simulink model "receiver_1"  (R2023a)
settings: Solver=FixedStepAuto  StartTime=0.0  StopTime=10.0  RelTol=1e-3
undefined symbols (not defined in the file): Data_Display, M, receiver_nihar, SC_1_DC_0
libraries: androiduilib x5, androidaudiovideolib x2, androidcommunicationlib x2
settings Model: Creator=mohit  LastModifiedBy=mohit
settings OptimizationCC: EnhancedBackFolding=on  PassReuseOutputArgsAs=Individual arguments  ZeroExternalMemoryAtStartup=off  ZeroInternalMemoryAtStartup=off  MaxStackSize=64  OptimizeBlockOrder=speed  DifferentSizesBufferReuse=on  OptimizationCustomize=off  EfficientTunableParamExpr=on
settings DebuggingCC: ParameterTunabilityLossMsg=error
settings HardwareCC: ProdBitPerLong=64  ProdLargestAtomicInteger=LongLong  ProdLargestAtomicFloat=Double  ProdLongLongMode=on  ProdHWDeviceType=ARM Compatible->ARM 64-bit (LP64)  UseEmbeddedCoderFeatures=off  UseSimulinkCoderFeatures=off
settings SFSimCC: MATLABDynamicMemAlloc=off
settings RTWCC: Description=Embedded Coder  SystemTargetFile=ert.tlc  HardwareBoard=Android Device (64bit)  TLCOptions="-aInlineSetEventsForThisBaseRateFcn=TLC_FALSE -aSuppressMultiTaskScheduler=TLC_FALSE  -aRateBasedStepFcn=0"  TemplateMakefile=ert_default_tmf  RTWVerbose=off  Toolchain=Android SDK/NDK Tools
settings CodeAppCC: ForceParamTrailComments=on  IgnoreCustomStorageClasses=off  OperatorAnnotations=on  SimulinkDataObjDesc=on  SFDataObjDesc=on  InsertBlockDesc=on
settings ERTTargetCC: SupportNonInlinedSFcns=on

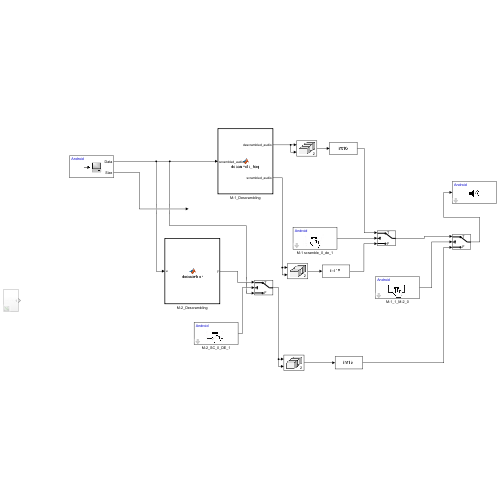
[thumbnail: Simulink's stored preview of the top-level diagram]
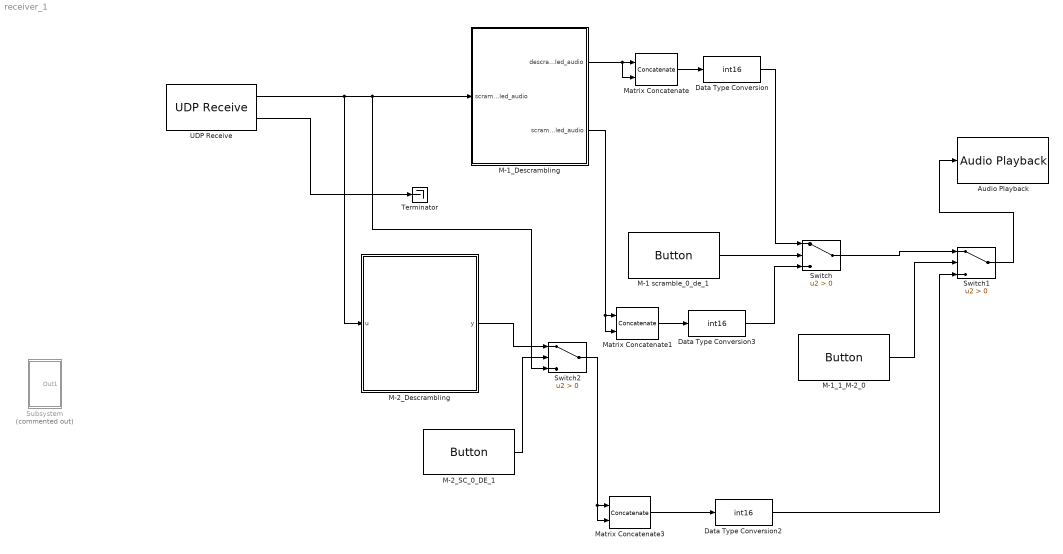
== system receiver_1 ==
  Audio Playback : androidaudiovideolib/Audio Playback  SampleFreq=44100  AudioSamplingFreq=44100  SampleTime=0.1  DeviceStr=0  QueueDuration=0  BlockPlatform=Android
  Data Type Conversion : DataTypeConversion  OutDataTypeStr=int16  SaturateOnIntegerOverflow=off  RndMeth=Floor
  Data Type Conversion2 : DataTypeConversion  OutDataTypeStr=int16  SaturateOnIntegerOverflow=off  RndMeth=Floor
  Data Type Conversion3 : DataTypeConversion  OutDataTypeStr=int16  SaturateOnIntegerOverflow=off  RndMeth=Floor
  M-1 scramble_0_de_1 : androiduilib/Button  ButtonState=Not pressed  ButtonId=receiver_nihar/M-1_scramble_0_de_1  State=off  SampleTime=0.1  BlockPlatform=Android
  M-1_1_M-2_0 : androiduilib/Button  ButtonState=Not pressed  ButtonId=receiver_nihar/M-1_1_M-2_0  State=off  SampleTime=0.1  BlockPlatform=Android
  M-1_Descrambling : MATLAB Function  TreatAsAtomicUnit=on
  M-2_Descrambling : MATLAB Function  TreatAsAtomicUnit=on
  M-2_SC_0_DE_1 : androiduilib/Button  ButtonState=Not pressed  ButtonId=receiver_nihar/M-2_SC_0_DE_1  State=off  SampleTime=0.1  BlockPlatform=Android
  Matrix Concatenate : Concatenate  Mode=Multidimensional array  ConcatenateDimension=2
  Matrix Concatenate1 : Concatenate  Mode=Multidimensional array  ConcatenateDimension=2
  Matrix Concatenate3 : Concatenate  Mode=Multidimensional array  ConcatenateDimension=2
  Subsystem : Subsystem  Commented=on
  Switch : Switch  Criteria=u2 > Threshold  SaturateOnIntegerOverflow=off  InputSameDT=off
  Switch1 : Switch  Criteria=u2 > Threshold  SaturateOnIntegerOverflow=off  InputSameDT=off
  Switch2 : Switch  Criteria=u2 > Threshold  SaturateOnIntegerOverflow=off  InputSameDT=off
  Terminator : Terminator
  UDP Receive : androidcommunicationlib/UDP Receive  localURL='0.0.0.0'  localPort=35000  remoteURL='0.0.0.0'  remotePort=-1  recvBufferSize=8192  signalDatatype=int16  dims=2205  isVarSize=off  showBlockingTime=off  blockingTime=0  sampletime=0.05  blockPlatform=Android
  wires:
  UDP Receive/2 -> Terminator/1
  M-1_Descrambling/1(descrambled_audio) -> Matrix Concatenate/2, Matrix Concatenate/1
  Matrix Concatenate/1 -> Data Type Conversion/1
  M-1 scramble_0_de_1/1 -> Switch/2
  UDP Receive/1 -> Switch2/3, M-1_Descrambling/1("scrambled_audio "), M-2_Descrambling/1(u)
  M-1_Descrambling/2(scrambled_audio) -> Matrix Concatenate1/2, Matrix Concatenate1/1
  Data Type Conversion/1 -> Switch/1
  Matrix Concatenate3/1 -> Data Type Conversion2/1
  Matrix Concatenate1/1 -> Data Type Conversion3/1
  Data Type Conversion3/1 -> Switch/3
  Switch/1 -> Switch1/1
  Switch1/1 -> Audio Playback/1
  M-1_1_M-2_0/1 -> Switch1/2
  M-2_Descrambling/1(y) -> Switch2/1
  M-2_SC_0_DE_1/1 -> Switch2/2
  Switch2/1 -> Matrix Concatenate3/2, Matrix Concatenate3/1
  Data Type Conversion2/1 -> Switch1/3

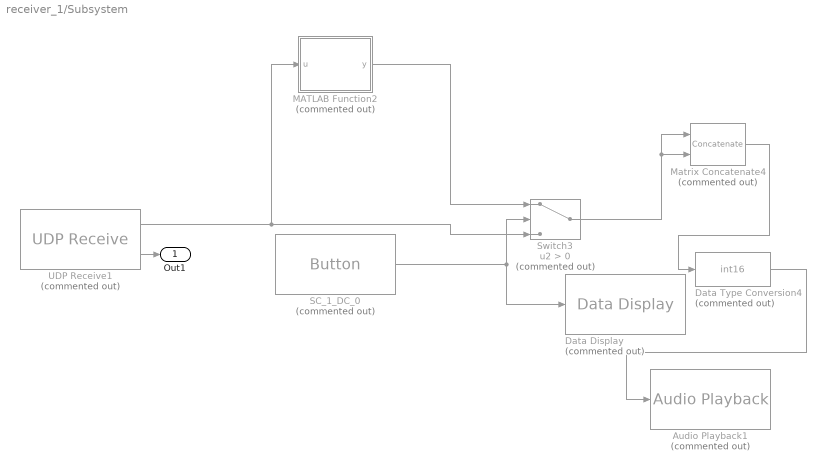
== system receiver_1/Subsystem ==
  Audio Playback1 : androidaudiovideolib/Audio Playback  Commented=on  SampleFreq=44100  AudioSamplingFreq=44100  SampleTime=0.1  DeviceStr=0  QueueDuration=0  BlockPlatform=Android
  Data Display : androiduilib/Data Display  Commented=on  DataDisplayId=receiver_nihar/Data_Display  Format=Float  Precision=6  SimulateUsing=Code generation  blockPlatform=Android
  Data Type Conversion4 : DataTypeConversion  Commented=on  OutDataTypeStr=int16  SaturateOnIntegerOverflow=off  RndMeth=Floor
  MATLAB Function2 : MATLAB Function  Commented=on  TreatAsAtomicUnit=on
  Matrix Concatenate4 : Concatenate  Commented=on  Mode=Multidimensional array  ConcatenateDimension=2
  SC_1_DC_0 : androiduilib/Button  Commented=on  ButtonState=Not pressed  ButtonId=receiver_nihar/SC_1_DC_0  State=off  SampleTime=0.1  BlockPlatform=Android
  Switch3 : Switch  Commented=on  Criteria=u2 > Threshold  SaturateOnIntegerOverflow=off  InputSameDT=off
  UDP Receive1 : androidcommunicationlib/UDP Receive  Commented=on  localURL='0.0.0.0'  localPort=35000  remoteURL='0.0.0.0'  remotePort=-1  recvBufferSize=8192  signalDatatype=int16  dims=2205  isVarSize=off  showBlockingTime=off  blockingTime=0  sampletime=0.05  blockPlatform=Android
  Out1 : Outport
  wires:
  Data Type Conversion4/1 -> Audio Playback1/1
  Switch3/1 -> Matrix Concatenate4/1, Matrix Concatenate4/2
  SC_1_DC_0/1 -> Data Display/1, Switch3/2
  UDP Receive1/1 -> Switch3/3, MATLAB Function2/1(u)
  UDP Receive1/2 -> Out1/1
  Matrix Concatenate4/1 -> Data Type Conversion4/1
  MATLAB Function2/1(y) -> Switch3/1

== matlab function receiver_1/M-2_Descrambling ==
  data: u input; y output
function y = descrambler(u)
    % Extract the first channel of the input matrix (assuming u is Nx2)
    u = u(:,1);

    % Define the bucket size
    bucketSize = 20;

    % Perform FFT on the entire signal
    fftResult = fft(u);
    
    % Number of buckets in the entire signal
    numBuckets = floor(length(fftResult) / bucketSize);

    % Subtract the exact noise added during scrambling
    for i = 1:numBuckets
        % Define the range of indices for this bucket
        bucketStartIdx = (i-1) * bucketSize + 1;
        bucketEndIdx = bucketStartIdx + bucketSize - 1;

        % Remove noise from each element in the bucket
        for idx = bucketStartIdx:bucketEndIdx
            noise = (idx +10) * 1e6;  % Calculate noise as index * 10,00,000
            fftResult(idx) = fftResult(idx) - noise;  % Remove noise from positive frequency
            fftResult(end - idx + 2) = fftResult(end - idx + 2) - noise;  % Remove noise from negative frequency
        end
    end

    % Handle any remaining elements outside of full buckets
    if mod(length(fftResult), bucketSize) ~= 0
        remainingStart = numBuckets * bucketSize + 1;
        for idx = remainingStart:length(fftResult)
            noise = (idx+10) * 1e6;  % Calculate noise as index * 10,00,000
            fftResult(idx) = fftResult(idx) - noise;  % Remove noise from positive frequency
            fftResult(end - idx + 2) = fftResult(end - idx + 2) - noise;  % Remove noise from negative frequency
        end
    end

    % Enforce conjugate symmetry on fftResult to ensure real output from ifft
    N = length(fftResult);
    fftResult(2:N/2) = conj(fftResult(N:-1:N/2+2));

    % Perform the inverse FFT to get the descrambled time-domain signal
    descrambledChannel = ifft(fftResult);

    % Take the real part to ensure the output is real-valued
    y = real(descrambledChannel);
end

== matlab function receiver_1/M-1_Descrambling ==
  data: scrambled_audio input; descrambled_audio output; scrambled_audio output
function [descrambled_audio,scrambled_audio] = descramble_freq(scrambled_audio)
    % Descramble the scrambled audio input in the frequency domain using the same seed
    % scrambled_audio: [nx2] scrambled audio array
    % seed: The same integer seed used during scrambling
    seed=123;
    % Pre-allocate descrambled_audio array
    descrambled_audio = zeros(size(scrambled_audio));

    % Set the random seed to regenerate the same permutation
    rng(seed, 'twister');
    
    % Generate the same random permutation as scrambling
    n = size(scrambled_audio, 1);
    swap_indices = randperm(n);
    scrambled_audio=scrambled_audio(:,1);
    % Apply FFT to each channel separately
    scrambled_freq_left = fft(scrambled_audio(:,1));
    %scrambled_freq_right = fft(scrambled_audio(:,2));

    % Reverse the swapping using the inverse of swap_indices
    [~, inverse_indices] = sort(swap_indices);
    descrambled_freq_left = scrambled_freq_left(inverse_indices);
    %descrambled_freq_right = scrambled_freq_right(inverse_indices);

    % Convert back to time domain
    descrambled_audio(:,1) = real(ifft(descrambled_freq_left));
    %descrambled_audio(:,2) = real(ifft(descrambled_freq_right));
end

== matlab function receiver_1/Subsystem/MATLAB Function2 ==
  data: u input; y output
function y = descrambler(u)
    % Extract the first channel of the input matrix (assuming u is Nx2)
    u = u(:,1);

    % Define the bucket size
    bucketSize = 20;

    % Perform FFT on the entire signal
    fftResult = fft(u);
    
    % Number of buckets in the entire signal
    numBuckets = floor(length(fftResult) / bucketSize);

    % Subtract the exact noise added during scrambling
    for i = 1:numBuckets
        % Define the range of indices for this bucket
        bucketStartIdx = (i-1) * bucketSize + 1;
        bucketEndIdx = bucketStartIdx + bucketSize - 1;

        % Remove noise from each element in the bucket
        for idx = bucketStartIdx:bucketEndIdx
            noise = (idx +10) * 1e6;  % Calculate noise as index * 10,00,000
            fftResult(idx) = fftResult(idx) - noise;  % Remove noise from positive frequency
            fftResult(end - idx + 2) = fftResult(end - idx + 2) - noise;  % Remove noise from negative frequency
        end
    end

    % Handle any remaining elements outside of full buckets
    if mod(length(fftResult), bucketSize) ~= 0
        remainingStart = numBuckets * bucketSize + 1;
        for idx = remainingStart:length(fftResult)
            noise = (idx+10) * 1e6;  % Calculate noise as index * 10,00,000
            fftResult(idx) = fftResult(idx) - noise;  % Remove noise from positive frequency
            fftResult(end - idx + 2) = fftResult(end - idx + 2) - noise;  % Remove noise from negative frequency
        end
    end

    % Enforce conjugate symmetry on fftResult to ensure real output from ifft
    N = length(fftResult);
    fftResult(2:N/2) = conj(fftResult(N:-1:N/2+2));

    % Perform the inverse FFT to get the descrambled time-domain signal
    descrambledChannel = ifft(fftResult);

    % Take the real part to ensure the output is real-valued
    y = real(descrambledChannel);
end
